simulink subsystem "Torque_Vectoring"  (R2023b)
settings: Solver=VariableStepAuto  StartTime=0.0  StopTime=10.0  RelTol=1e-3
undefined symbols (not defined in the file): chassis, powertrain, suspension, tvs
libraries: simulink x1
settings Model: Creator=Inver  LastModifiedBy=Inver
settings SFSimCC: SimCustomHeaderCode="#include \"simplex.h\""  SimUserSources=Code_Generation_Project/simplex.c

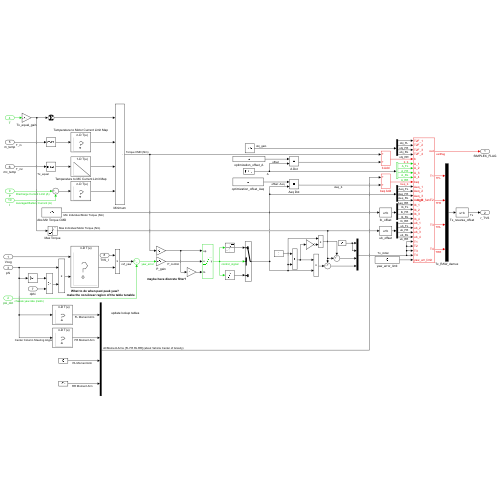
[thumbnail: Simulink's stored preview of the top-level diagram]
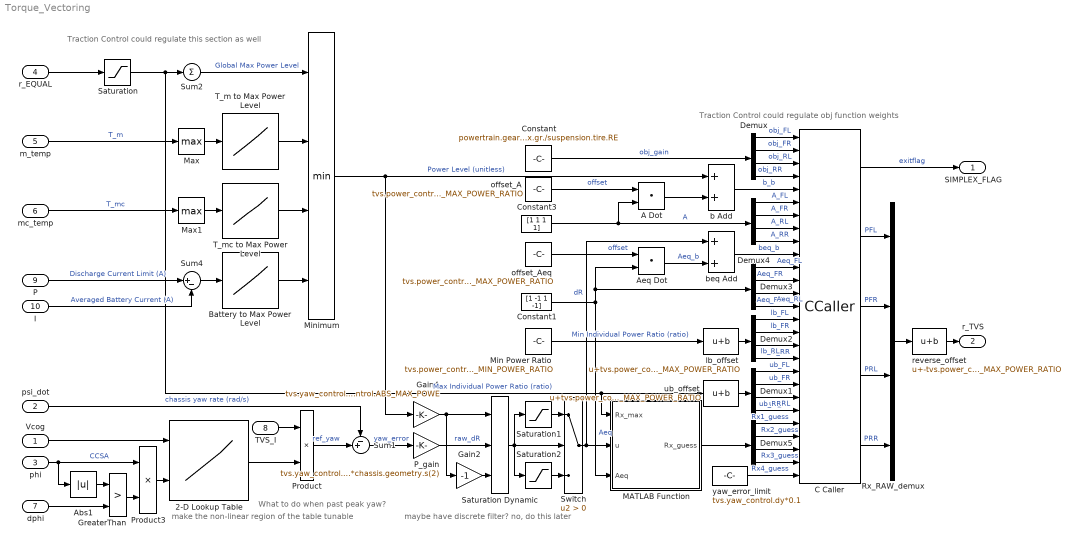
== system Torque_Vectoring ==
  note: What to do when past peak yaw?
  note: maybe have discrete filter? no, do this later
  note: make the non-linear region of the table tunable
  note: Traction Control could regulate this section as well
  note: Traction Control could regulate obj function weights
  Vcog : Inport
  psi_dot : Inport  Port=2  OutDataTypeStr=double  LockScale=on
  phi : Inport  Port=3
  r_EQUAL : Inport  Port=4  OutDataTypeStr=double  LockScale=on
  m_temp : Inport  Port=5
  mc_temp : Inport  Port=6
  dphi : Inport  Port=7
  TVS_I : Inport  Port=8
  P : Inport  Port=9  OutDataTypeStr=double  LockScale=on
  I : Inport  Port=10  OutDataTypeStr=double  LockScale=on
  2-D Lookup Table : Lookup_n-D  BreakpointsForDimension1=tvs.yaw_control.max_v_bp(1:34)  BreakpointsForDimension2=[-fliplr(tvs.yaw_control.max_s_bp(2:end)) tvs.yaw_control.max_s_bp]  Table=[-flipud(tvs.yaw_control.max_yaw_table_ref(2:end,1:34)); tvs.yaw_control.max_yaw_table_ref(:,1:34)]'  ExtrapMethod=Clip  InternalRulePriority=Speed  RndMeth=Simplest
      settings: InputPortMap=u0,u1
  A Dot : DotProduct  OutDataTypeStr=double
  Abs1 : Abs  SaturateOnIntegerOverflow=off
  Aeq Dot : DotProduct  OutDataTypeStr=double
  Battery to Max Power Level : Lookup_n-D  NumberOfTableDimensions=1  LookupTableObject=''  BreakpointsForDimension1=[0 5]  BreakpointsForDimension1FirstPoint=10  BreakpointsForDimension2FirstPoint=10  BreakpointsForDimension1Spacing=12  BreakpointsForDimension2Spacing=12  IndexSearchMethod=Evenly spaced points  Table=[0 tvs.power_control.ABS_MAX_POWER_LEVEL]  ExtrapMethod=Clip  InternalRulePriority=Speed  RndMeth=Simplest
  C Caller : CCaller  FunctionName=bigM_func
  Constant : Constant  Value=powertrain.gearbox.gr./suspension.tire.RE
  Constant1 : Constant  Value=[1 -1 1 -1]
  Constant3 : Constant  Value=[1 1 1 1]
  Demux{,1..5} (6 alike) : Demux
  Gain2 : Gain  Gain=-1
  Gain4 : Gain  Gain=tvs.yaw_control.power_sat_const/tvs.power_control.ABS_MAX_POWE
  GreaterThan : RelationalOperator  Operator=>  OutDataTypeStr=boolean  RndMeth=Simplest  InputSameDT=off
  MATLAB Function : MATLAB Function  TreatAsAtomicUnit=on
  Max : MinMax  Function=max
  Max1 : MinMax  Function=max
  Min Power Ratio : Constant  Value=tvs.power_control.ABS_MIN_POWER_RATIO  OutDataTypeStr=double
  Minimum : MinMax  Inputs=4
  P_gain : Gain  Gain=tvs.yaw_control.P*chassis.geometry.s(2)  ParamDataTypeStr=double  OutDataTypeStr=double
  Product : Product  OutDataTypeStr=Inherit: Inherit via back propagation
  Product3 : Product
  Rx_RAW_demux : Mux
  Saturation : Saturate  UpperLimit=tvs.power_control.ABS_MAX_POWER_RATIO  LowerLimit=2.*tvs.power_control.dRx  OutDataTypeStr=Inherit: Inherit via back propagation
  Saturation Dynamic : simulink/Discontinuities/Saturation Dynamic  OutMin=[]  OutMax=[]  OutDataTypeStr=Inherit: Same as second input  OutDataType=fixdt(1, 16)  OutScaling=2^-10  DoSatur=off
  Saturation1 : Saturate  UpperLimit=inf  LowerLimit=tvs.yaw_control.dB
  Saturation2 : Saturate  UpperLimit=-tvs.yaw_control.dB  LowerLimit=-inf
  Sum1 : Sum  Inputs=-+|  OutDataTypeStr=Inherit: Inherit via back propagation
  Sum2 : Sum  Inputs=+
  Sum4 : Sum  Inputs=|+-
  Switch : Switch  Criteria=u2 > Threshold  SaturateOnIntegerOverflow=off  InputSameDT=off
  T_m to Max Power Level : Lookup_n-D  NumberOfTableDimensions=1  BreakpointsForDimension1=tvs.power_control.motor_t_bp  IndexSearchMethod=Evenly spaced points  Table=[tvs.power_control.ABS_MAX_POWER_LEVEL 0]  ExtrapMethod=Clip  UseLastTableValue=on  InternalRulePriority=Speed  RndMeth=Simplest
  T_mc to Max Power Level : Lookup_n-D  NumberOfTableDimensions=1  BreakpointsForDimension1=[50 75]  IndexSearchMethod=Evenly spaced points  Table=[tvs.power_control.ABS_MAX_POWER_LEVEL 0]  ExtrapMethod=Clip  UseLastTableValue=on  InternalRulePriority=Speed  RndMeth=Simplest
  b Add : Sum  OutDataTypeStr=double
  beq Add : Sum  OutDataTypeStr=double
  lb_offset : Bias  Bias=tvs.power_control.ABS_MAX_POWER_RATIO  SaturateOnIntegerOverflow=off
  offset_A : Constant  Value=tvs.power_control.ABS_MAX_POWER_RATIO  OutDataTypeStr=double
  offset_Aeq : Constant  Value=tvs.power_control.ABS_MAX_POWER_RATIO  OutDataTypeStr=double
  reverse_offset : Bias  Bias=-tvs.power_control.ABS_MAX_POWER_RATIO  SaturateOnIntegerOverflow=off
  ub_offset : Bias  Bias=tvs.power_control.ABS_MAX_POWER_RATIO  SaturateOnIntegerOverflow=off
  yaw_error_limit : Constant  Value=tvs.yaw_control.dy*0.1  OutDataTypeStr=double
  SIMPLEX_FLAG : Outport
  r_TVS : Outport  Port=2
  wires:
  MATLAB Function/1(Rx_guess) -> Demux5/1
  Demux5/4 -> C Caller/26  "Rx4_guess"
  Demux5/3 -> C Caller/25  "Rx3_guess"
  Demux5/2 -> C Caller/24  "Rx2_guess"
  Demux5/1 -> C Caller/23  "Rx1_guess"
  Sum4/1 -> Battery to Max Power Level/1
  I/1 -> Sum4/2  "Averaged Battery Current (A)"
  Battery to Max Power Level/1 -> Minimum/4
  reverse_offset/1 -> r_TVS/1
  C Caller/1 -> SIMPLEX_FLAG/1  "exitflag"
  P/1 -> Sum4/1  "Discharge Current Limit (A)"
  Product3/1 -> 2-D Lookup Table/2
  Sum2/1 -> Minimum/1  "Global Max Power Level"
  phi/1 -> Product3/1, Abs1/1  "CCSA"
  Rx_RAW_demux/1 -> reverse_offset/1
  r_EQUAL/1 -> Saturation/1
  Demux/2 -> C Caller/2  "obj_FR"
  Switch/1 -> beq Add/1, MATLAB Function/2(u)  "dR"
  Demux/4 -> C Caller/4  "obj_RR"
  Demux4/3 -> C Caller/8  "A_RL"
  offset_A/1 -> A Dot/1  "offset"
  Demux/3 -> C Caller/3  "obj_RL"
  Demux1/1 -> C Caller/19  "ub_FL"
  Demux4/1 -> C Caller/6  "A_FL"
  Demux1/2 -> C Caller/20  "ub_FR"
  ub_offset/1 -> Demux1/1
  b Add/1 -> C Caller/5  "b_b"
  Demux1/3 -> C Caller/21  "ub_RL"
  C Caller/3 -> Rx_RAW_demux/2  "PFR"
  Demux4/4 -> C Caller/9  "A_RR"
  Aeq Dot/1 -> beq Add/2  "Aeq_b"
  Demux3/4 -> C Caller/14  "Aeq_RR"
  C Caller/2 -> Rx_RAW_demux/1  "PFL"
  C Caller/4 -> Rx_RAW_demux/3  "PRL"
  offset_Aeq/1 -> Aeq Dot/1  "offset"
  Demux/1 -> C Caller/1  "obj_FL"
  Demux2/2 -> C Caller/16  "lb_FR"
  Constant3/1 -> Demux4/1, A Dot/2  "A"
  C Caller/5 -> Rx_RAW_demux/4  "PRR"
  Demux3/2 -> C Caller/12  "Aeq_FR"
  Demux2/1 -> C Caller/15  "lb_FL"
  yaw_error_limit/1 -> C Caller/27
  Constant/1 -> Demux/1  "obj_gain"
  lb_offset/1 -> Demux2/1
  Demux1/4 -> C Caller/22  "ub_RR"
  A Dot/1 -> b Add/2
  Demux4/2 -> C Caller/7  "A_FR"
  Demux2/4 -> C Caller/18  "lb_RR"
  Demux3/3 -> C Caller/13  "Aeq_RL"
  Demux3/1 -> C Caller/11  "Aeq_FL"
  Demux2/3 -> C Caller/17  "lb_RL"
  beq Add/1 -> C Caller/10  "beq_b"
  m_temp/1 -> Max/1  "T_m"
  Saturation/1 -> MATLAB Function/1(Rx_max), ub_offset/1, Sum2/1  "Max Individual Power Ratio (ratio)"
  Min Power Ratio/1 -> lb_offset/1  "Min Individual Power Ratio (ratio)"
  Minimum/1 -> Gain4/1, b Add/1  "Power Level (unitless)"
  Vcog/1 -> 2-D Lookup Table/1
  mc_temp/1 -> Max1/1  "T_mc"
  Max1/1 -> T_mc to Max Power Level/1
  T_m to Max Power Level/1 -> Minimum/2
  T_mc to Max Power Level/1 -> Minimum/3
  Max/1 -> T_m to Max Power Level/1
  TVS_I/1 -> Product/1
  Product/1 -> Sum1/2  "ref_yaw"
  psi_dot/1 -> Sum1/1  "chassis yaw rate (rad/s)"
  Saturation Dynamic/1 -> Switch/2, Saturation1/1, Saturation2/1
  2-D Lookup Table/1 -> Product/2
  GreaterThan/1 -> Product3/2
  Abs1/1 -> GreaterThan/1
  Saturation1/1 -> Switch/1
  Sum1/1 -> P_gain/1  "yaw_error"
  Gain2/1 -> Saturation Dynamic/3
  Saturation2/1 -> Switch/3
  Gain4/1 -> Saturation Dynamic/1, Gain2/1
  dphi/1 -> GreaterThan/2
  P_gain/1 -> Saturation Dynamic/2  "raw_dR"
  Constant1/1 -> MATLAB Function/3(Aeq), Demux3/1, Aeq Dot/2  "Aeq"

== matlab function Torque_Vectoring/MATLAB Function ==
  data: Rx_max input; u input; Aeq input; Rx_guess output; tvs parameter
function Rx_guess = compute_tx_guess(Rx_max,u,Aeq, tvs)
    if u > 0
        Rx_guess = [0 0 Rx_max(3) Rx_max(4) - abs(u/Aeq(3))] + tvs.power_control.ABS_MAX_POWER_RATIO;
    else
        Rx_guess = [0 0 Rx_max(3) - abs(u/Aeq(3)) Rx_max(4)] + tvs.power_control.ABS_MAX_POWER_RATIO;
    end
end
